simulink library "LinkLibrary"  (R2022b)
settings: Solver=VariableStepAuto  StartTime=0.0  StopTime=10.0  RelTol=1e-3
libraries: arduinolib x5, simulink_extras x4, $bdroot x4, arduinosensorlib x1
settings Model: Creator=marti  LastModifiedBy=marti

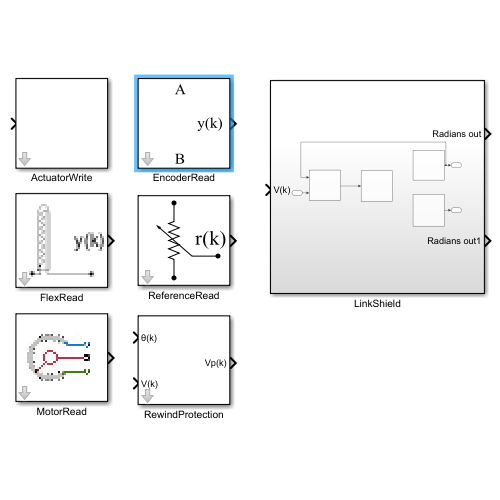
[thumbnail: Simulink's stored preview of the top-level diagram]
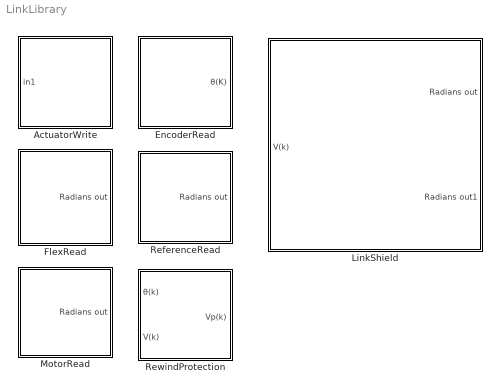
== system LinkLibrary ==
  ActuatorWrite : Subsystem
      mask Display: image('assets/LinkFig/Motor.svg');
  EncoderRead : Subsystem  mask{EncoderResolution=6, GearRation=120}
      mask prompts: EncoderResolution "Encoder Resolution"; GearRation "Gear Ration"
      mask DialogControl DescGroupVar Prompt: Encoder Read
      mask DialogControl DescTextVar Prompt: The block read position from incremental encoder and store position in incremental tics count. Than the incremental value is converted to radians. Before starting the program, it is necessary to turn the motor shaft to the zero position or perform a calibration. For proper operation on most Arduino boards use pins 2 and 3. Be careful with timer selection when using with sampling.
      mask Display: image('$imagefile'); % Use "Edit Image" on toolstrip to change.
  FlexRead : Subsystem
  LinkShield : Subsystem
  MotorRead : Subsystem
  ReferenceRead : Subsystem
      mask Display: image('assets/Potentiometer.svg');
  RewindProtection : Subsystem
      mask DialogControl DescGroupVar Prompt: RewindProtection
      mask DialogControl DescTextVar Prompt: The block shutdown input if the motor ange is more than maximal value.

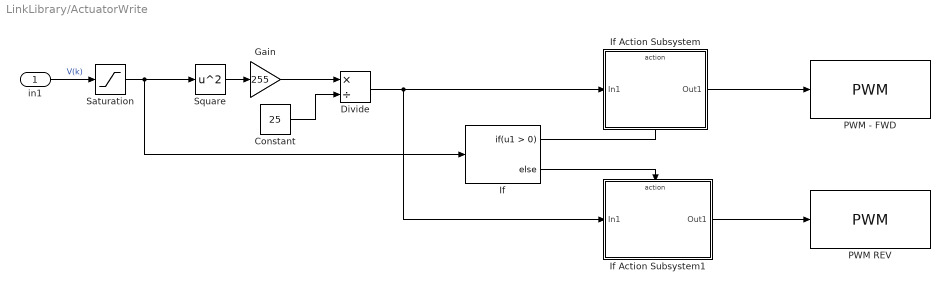
== system LinkLibrary/ActuatorWrite ==
  in1 : Inport
  Constant : Constant  Value=25
  Divide : Product  Inputs=*/
  Gain : Gain  Gain=255
  If : If
  If Action Subsystem : Subsystem  TreatAsAtomicUnit=on
  If Action Subsystem1 : Subsystem  TreatAsAtomicUnit=on
  PWM - FWD : arduinolib/PWM  pinNumber=5  frequencyType=Default  desiredFrequency=490.2  achievableFrequency=490.2
  PWM REV : arduinolib/PWM  pinNumber=6  frequencyType=Default  desiredFrequency=490.2  achievableFrequency=490.2
  Saturation : Saturate  UpperLimit=5  LowerLimit=-5
  Square : Math  Operator=square
  wires:
  If Action Subsystem1/1(Out1) -> PWM REV/1
  If/2 -> If Action Subsystem1/Action
  If/1 -> If Action Subsystem/Action
  If Action Subsystem/1(Out1) -> PWM - FWD/1
  Divide/1 -> If Action Subsystem1/1(In1), If Action Subsystem/1(In1)
  Constant/1 -> Divide/2
  Gain/1 -> Divide/1
  Square/1 -> Gain/1
  in1/1 -> Saturation/1  "V(k)"
  Saturation/1 -> Square/1, If/1

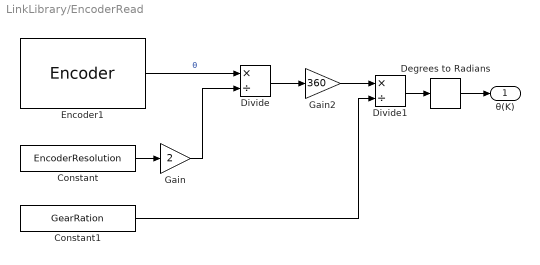
== system LinkLibrary/EncoderRead ==
  Constant : Constant  Value=EncoderResolution
  Constant1 : Constant  Value=GearRation
  Degrees to Radians : simulink_extras/Transformations/Degrees to Radians
  Divide : Product  Inputs=*/
  Divide1 : Product  Inputs=*/
  Encoder1 : arduinosensorlib/Encoder  InputA=2  InputB=3  Mode=No reset  SampleTime=-1
  Gain : Gain  Gain=2
  Gain2 : Gain  Gain=360
  θ(K) : Outport
  wires:
  Encoder1/1 -> Divide/1  "θ"
  Constant/1 -> Gain/1
  Gain/1 -> Divide/2
  Divide/1 -> Gain2/1
  Divide1/1 -> Degrees to Radians/1
  Gain2/1 -> Divide1/1
  Constant1/1 -> Divide1/2
  Degrees to Radians/1 -> θ(K)/1

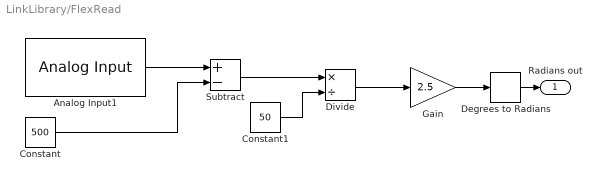
== system LinkLibrary/FlexRead ==
  Analog Input1 : arduinolib/Analog Input  pinNumber=1  ReadResultsOnly=off  ConversionTriggerSource=Software  ExternalTriggerType=uint32( 0 )  OutputDataType=uint16  EnableConversionCompleteNotify=off  EnableOuputStatus=off  SampleTime=-1  blockPlatform=arduino
  Constant : Constant  Value=500
  Constant1 : Constant  Value=50
  Degrees to Radians : simulink_extras/Transformations/Degrees to Radians
  Divide : Product  Inputs=*/
  Gain : Gain  Gain=2.5
  Subtract : Sum  Inputs=+-
  Radians out : Outport
  wires:
  Constant/1 -> Subtract/2
  Analog Input1/1 -> Subtract/1
  Gain/1 -> Degrees to Radians/1
  Constant1/1 -> Divide/2
  Divide/1 -> Gain/1
  Subtract/1 -> Divide/1
  Degrees to Radians/1 -> Radians out/1

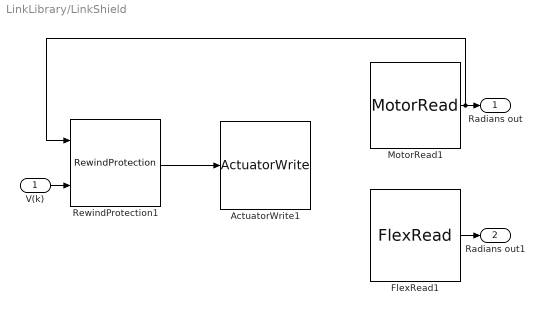
== system LinkLibrary/LinkShield ==
  V(k) : Inport
  ActuatorWrite1 : $bdroot/ActuatorWrite
  FlexRead1 : $bdroot/FlexRead
  MotorRead1 : $bdroot/MotorRead
  RewindProtection1 : $bdroot/RewindProtection
  Radians out : Outport
  Radians out1 : Outport  Port=2
  wires:
  RewindProtection1/1 -> ActuatorWrite1/1
  MotorRead1/1 -> RewindProtection1/1, Radians out/1
  V(k)/1 -> RewindProtection1/2
  FlexRead1/1 -> Radians out1/1

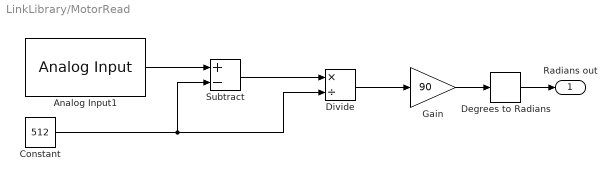
== system LinkLibrary/MotorRead ==
  Analog Input1 : arduinolib/Analog Input  pinNumber=2  ReadResultsOnly=off  ConversionTriggerSource=Software  ExternalTriggerType=uint32( 0 )  OutputDataType=uint16  EnableConversionCompleteNotify=off  EnableOuputStatus=off  SampleTime=-1  blockPlatform=arduino
  Constant : Constant  Value=512
  Degrees to Radians : simulink_extras/Transformations/Degrees to Radians
  Divide : Product  Inputs=*/
  Gain : Gain  Gain=90
  Subtract : Sum  Inputs=+-
  Radians out : Outport
  wires:
  Constant/1 -> Divide/2, Subtract/2
  Gain/1 -> Degrees to Radians/1
  Subtract/1 -> Divide/1
  Analog Input1/1 -> Subtract/1
  Divide/1 -> Gain/1
  Degrees to Radians/1 -> Radians out/1

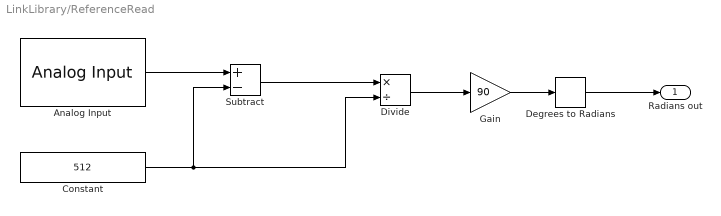
== system LinkLibrary/ReferenceRead ==
  Analog Input : arduinolib/Analog Input  pinNumber=0  ReadResultsOnly=off  ConversionTriggerSource=Software  ExternalTriggerType=uint32( 0 )  OutputDataType=uint16  EnableConversionCompleteNotify=off  EnableOuputStatus=off  SampleTime=-1  blockPlatform=arduino
  Constant : Constant  Value=512
  Degrees to Radians : simulink_extras/Transformations/Degrees to Radians
  Divide : Product  Inputs=*/
  Gain : Gain  Gain=90
  Subtract : Sum  Inputs=+-
  Radians out : Outport
  wires:
  Constant/1 -> Divide/2, Subtract/2
  Divide/1 -> Gain/1
  Analog Input/1 -> Subtract/1
  Degrees to Radians/1 -> Radians out/1
  Gain/1 -> Degrees to Radians/1
  Subtract/1 -> Divide/1

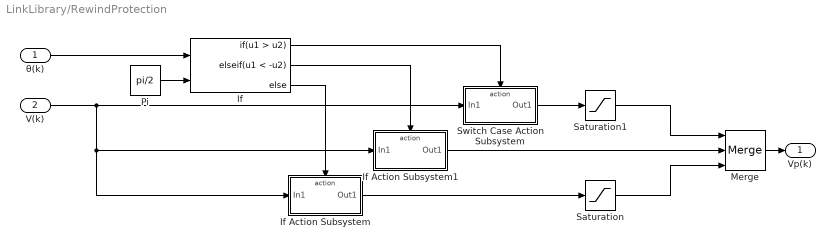
== system LinkLibrary/RewindProtection ==
  θ(k) : Inport
  V(k) : Inport  Port=2
  If : If  NumInputs=2  IfExpression=u1 > u2  ElseIfExpressions=u1 < -u2
  If Action Subsystem : Subsystem  TreatAsAtomicUnit=on
  If Action Subsystem1 : Subsystem  TreatAsAtomicUnit=on
  Merge : Merge  Inputs=3
  Pi : Constant  Value=pi/2  OutDataTypeStr=Inherit: Inherit via back propagation
  Saturation : Saturate  UpperLimit=5  LowerLimit=0
  Saturation1 : Saturate  UpperLimit=0  LowerLimit=-5
  Switch Case Action Subsystem : Subsystem  TreatAsAtomicUnit=on
  Vp(k) : Outport
  wires:
  If Action Subsystem1/1(Out1) -> Merge/2
  Switch Case Action Subsystem/1(Out1) -> Saturation1/1
  If/2 -> If Action Subsystem1/Action
  If/1 -> Switch Case Action Subsystem/Action
  Saturation1/1 -> Merge/1
  Saturation/1 -> Merge/3
  If Action Subsystem/1(Out1) -> Saturation/1
  V(k)/1 -> If Action Subsystem1/1(In1), If Action Subsystem/1(In1), Switch Case Action Subsystem/1(In1)
  If/3 -> If Action Subsystem/Action
  Merge/1 -> Vp(k)/1
  Pi/1 -> If/2
  θ(k)/1 -> If/1

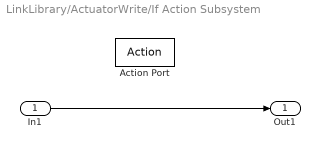
== system LinkLibrary/ActuatorWrite/If Action Subsystem ==
  In1 : Inport
  Action Port : ActionPort  ActionPortLabel=if(u1 > 0)
  Out1 : Outport
  wires:
  In1/1 -> Out1/1

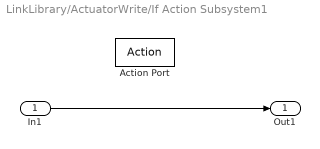
== system LinkLibrary/ActuatorWrite/If Action Subsystem1 ==
  In1 : Inport
  Action Port : ActionPort  ActionPortLabel=else
  Out1 : Outport
  wires:
  In1/1 -> Out1/1

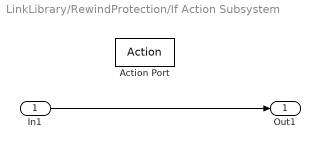
== system LinkLibrary/RewindProtection/If Action Subsystem ==
  In1 : Inport
  Action Port : ActionPort  ActionPortLabel=else
  Out1 : Outport
  wires:
  In1/1 -> Out1/1

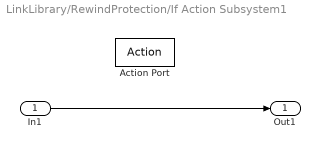
== system LinkLibrary/RewindProtection/If Action Subsystem1 ==
  In1 : Inport
  Action Port : ActionPort  ActionPortLabel=elseif(u1 < pi)
  Out1 : Outport
  wires:
  In1/1 -> Out1/1

== system LinkLibrary/RewindProtection/Switch Case Action Subsystem ==
  In1 : Inport
  Action Port : ActionPort  ActionPortLabel=if(u1 > pi)
  Out1 : Outport
  wires:
  In1/1 -> Out1/1
